simulink model "simulink_model"  (R2019a)
settings: Solver=VariableStepAuto  StartTime=0.0  StopTime=inf  RelTol=1e-3
libraries: dspnetwork x2, sldrtlib x1
settings Model: Creator=Admin  LastModifiedBy=Admin

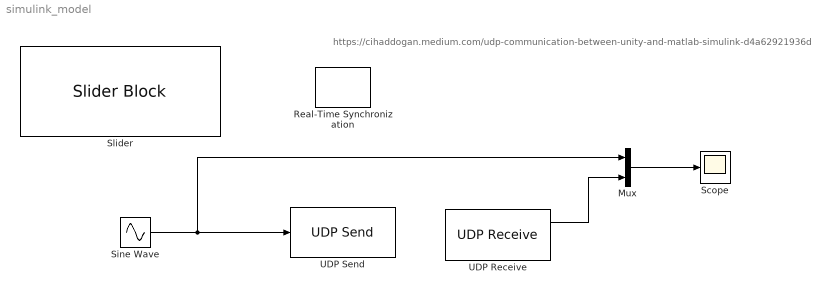
== system simulink_model ==
  note: https://cihaddogan.medium.com/udp-communication-between-unity-and-matlab-simulink-d4a62921936d
  Mux : Mux  Inputs=2
  Real-Time Synchronization : sldrtlib/Real-Time Synchronization  SampleTime=0.01  MaxMissedTicks=100000  ShowMissedTicks=off  YieldWhenWaiting=off
  Scope : Scope
  Sine Wave : Sin  Amplitude=61.76470588235294  Frequency=0.3  SampleTime=0
  Slider : SliderBlock
  UDP Receive : dspnetwork/UDP Receive  localURL='0.0.0.0'  localPort=26000  remoteURL='0.0.0.0'  remotePort=-1  recvBufferSize=8192  dims=255  signalDatatype=double  isComplex=off  isVarSize=off  showBlockingTime=off  blockingTime=0  sampletime=0.001  blockPlatform=[]
      settings: SourceProductName=Simulink
  UDP Send : dspnetwork/UDP Send  remoteURL='127.0.0.1'  remotePort=25000  localURL='0.0.0.0'  localPortSource=Automatically determine  localPort=-1  sampletime=-1  blockPlatform=[]  separateLengthPort=0
      settings: SourceProductName=Simulink
  wires:
  Mux/1 -> Scope/1
  Sine Wave/1 -> Mux/1, UDP Send/1
  UDP Receive/1 -> Mux/2
